simulink model "cubesatFullSim"  (R2024a)
settings: Solver=FixedStepAuto  StartTime=0.0  StopTime=20.0  FixedStep=0.1  MaxStep=1  MinStep=0.001  RelTol=1e-3
model workspace (MAT data in the model file):
  beta_initial = [0 0 0]
  com_quad_body = [1 0 0 0]
  imu_sample_time = 0.1
  initial_angular_momentum_body = [0 0 0]
  initial_datetime = [2020 3 17 23 48 32]
  initial_position_iss_orbit = [-2350000 -5230000 3530000]
  initial_quaterion_rotation = [0 0.7071 0.7071 0]
  initial_velocity_iss_orbit = [3990 -4820 -4820]
  intertia_tensor = [0.005743  -0.000107  -0.0006965; -0.000107  0.030927  8.6e-05; -0.000696  8.6e-05  0.030951]
  magnotorquer_current_to_magnetic = 1
  mass = 2.60014
  moi_spin_axis = 2.0292e-06
  onboard_att_ctrl_sample_time = 0.1
  onboard_att_det_sample_time = 0.1
  onboard_env_modelling_sample_time = 0.1
  q_n2m_initial = [1 0 0 0]
  reaction_wheel_state_space_A = [0  0  0  0; 0  0  0  0; 0  0  0  0; 0  0  0  0]
  reaction_wheel_state_space_B = [512  0  0  0; 0  512  0  0; 0  0  512  0; 0  0  0  512]
  reaction_wheel_state_space_C = [962.5  0  0  0; 0  962.5  0  0; 0  0  962.5  0; 0  0  0  962.5]
  reaction_wheel_state_space_D = [0  0  0  0; 0  0  0  0; 0  0  0  0; 0  0  0  0]
  reaction_wheel_state_space_initial = [0 0 0 0]
  steve_camera_axis_1 = [0 0 1]
  steve_camera_direction = [1 0 0]
libraries: vrlib x6
settings Model: Creator=samuel  LastModifiedBy=joshu
settings OptimizationCC: ReuseModelBlockBuffer=off
settings DebuggingCC: AlgebraicLoopMsg=error  ArtificialAlgebraicLoopMsg=error
settings ModelReferenceCC: EnableRefExpFcnMdlSchedulingChecks=on
settings RTWCC: GPUComputeCapability=3.5

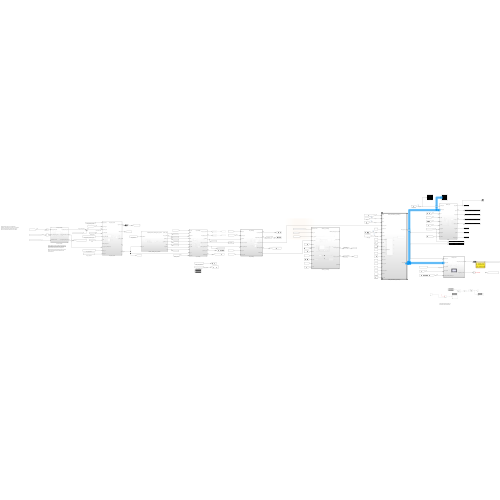
[thumbnail: Simulink's stored preview of the top-level diagram]
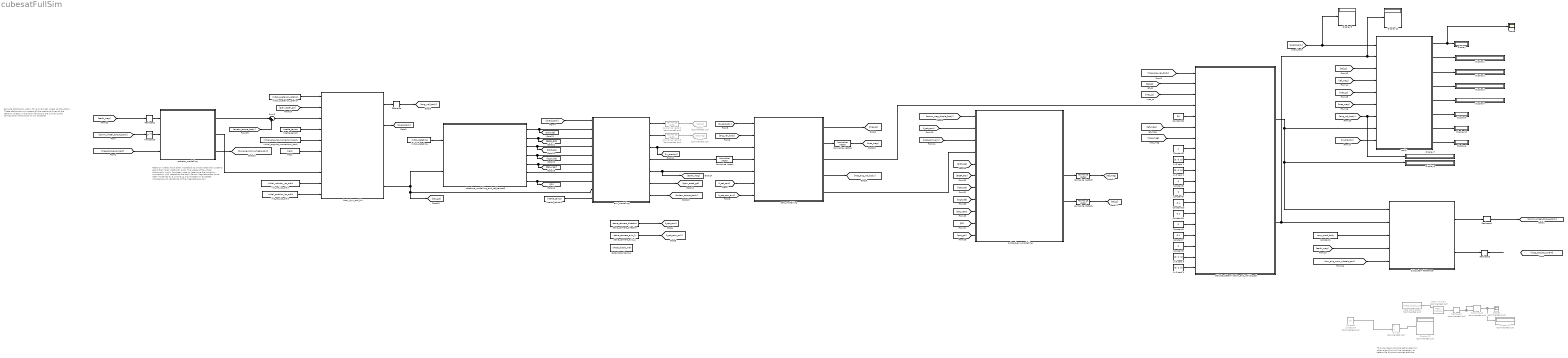
== system cubesatFullSim ==
  note: This provides a sample test quaternion, other algorithms will be necessary to determine this commanded attitude.
  note: Reaction wheels have been modelled as simple rotational systems about their local rotational axes. The usage of the wheel distribution matrix has been used to determine their angular momentum with respect to the body frame.
      |
      | Magnetorquers have been modelled as a simple LC circuit based on expected inductance and resistance of the magnetorquer coil.
  note: Sample distribution matrix for a pyramidal wheel configuration. These define the unit vectors of the rotational axes of the reaction wheels in the body frame and are similar to the configuration employed on our CubeSat.
  1x3 zero {1..4} (4 alike) : Constant  Value=[0, 0, 0]
  Constant : Constant  Commented=on  Value=2.0292e-6
  Constant1 : Constant  Value=com_quad_body
  Constant10 : Constant  Value=0.1
  Constant11 : Constant  Value=0.1
  Constant12 : Constant  Value=90
  Constant3 : Constant  OutDataTypeStr=boolean
  Constant5 : Constant  Value=0  OutDataTypeStr=boolean
  Constant6 : Constant  Value=0  OutDataTypeStr=boolean
  Constant7 : Constant  Value=0.1
  Constant8 : Constant  Value=0  OutDataTypeStr=boolean
  Constant9 : Constant  Value=0
  Data Store Memory : DataStoreMemory  DataStoreName=wheel_distrib_mat  WriteAfterWriteMsg=warning  InitialValue=[0.5736 0.5736 0.5736 0.5736 ; 0.8192 -0.8192 0 0 ; 0 0 0.8192 -0.8192]  ShowAdditionalParam=off
  Data Store Read1 : DataStoreRead  Commented=on  DataStoreName=wheel_distrib_mat  IndexOptions=Index vector (dialog)  Indices=1  OutputSizes=1
  Display{,1..11} (12 alike) : Display
  Display12 : Display  Commented=on
  Display13 : Display  Commented=on
  Divide : Product  Commented=on  Inputs=*/
  Dot Product : DotProduct  Commented=on  OutDataTypeStr=Inherit: Inherit via internal rule
  Goto7 : Goto  Commented=on  GotoTag=ref_ss
  Goto8 : Goto  Commented=on  GotoTag=ref_mag
  Matrix Multiply : Product  Commented=on  Multiplication=Matrix(*)
  Normalize Vector{,4..6} (4 alike) : vrlib/Utilities/Normalize Vector  maxzero=0
  Normalize Vector2 : vrlib/Utilities/Normalize Vector  Commented=on  maxzero=0
  Normalize Vector3 : vrlib/Utilities/Normalize Vector  Commented=on  maxzero=0
  Reshape : Reshape  OutputDimensionality=Row vector (2-D)
  Reshape1 : Reshape  OutputDimensionality=Row vector (2-D)
  Reshape2 : Reshape
  Reshape3 : Reshape
  Reshape5 : Reshape  Commented=on
  Scope : Scope
  Scope1 : Scope  Commented=on
  Subsystem Reference : Subsystem  TreatAsAtomicUnit=on  SystemSampleTime=onboard_att_ctrl_sample_time  ReferencedSubsystem=attitude_control
  Sum3 : Sum  Inputs=|++
  Transpose : Math  Operator=transpose
  Verify : Subsystem  ReferencedSubsystem=MEKF_verify
  actuator_modelling : Subsystem  ReferencedSubsystem=actuator_modelling
  attitude_determination_and_vehicle_est : Subsystem  TreatAsAtomicUnit=on  SystemSampleTime=onboard_att_det_sample_time  ReferencedSubsystem=attitude_determination_and_vehicle_est
      settings: PortSchema="{\"entries\":[{\"content\":{\"sides\":[{\"content\":{\"connectorIds\":[\"In1\",\"In2\",\"In3\",\"In4\",\"In15\",\"In5\",\"In6\",\"In7\",\"In8\",\"In9\",\"In10\",\"In11\",\"In12\",\"In13\",\"In14\",\"In16\",\"In17\",\"In18\",\"In19\"]},\"type\":\"ConnectorPlacement.EquallySpacedRectSide\",\"uuid\":\"3b22937b-158d-42bc-8266-221df4d5bb4f\"},{\"content\":{\"connectorIds\":[\"Out1\",\"Out2\"],\"side\":\"RIGHT\"},\"type\":\"ConnectorPlacement.EquallySpacedRectSide\",\"uuid\":\"2d7976b0-5d09-4ece-a5b5-6f5d6f0d46dd\"},{\"content\":{\"side\":\"TOP\"},\"type\":\"ConnectorPlacement.EquallySpacedRectSide\",\"uuid\":\"411abe81-91ab-4e83-a0ca-8600290f09f5\"}]},\"type\":\"ConnectorPlacement.EquallySpacedConnector\",\"uuid\":\"dff24d4c-a30b-41c1-92cc-a12930c50369\"}],\"packageUris\":[\"http://schema.mathworks.com/mf0/Connector/R2020b\"],\"version\":\"1.0\"}"
  body_dyn_and_kin : Subsystem  ReferencedSubsystem=body_dyn_and_kin
  datetime_modelling_and_ref_frames3 : Subsystem  ReferencedSubsystem=simplified_datetime_modelling_and_ref_frames
      settings: PortSchema="{\"entries\":[{\"content\":{\"sides\":[{\"content\":{\"connectorIds\":[\"In2\",\"In1\"]},\"type\":\"ConnectorPlacement.EquallySpacedRectSide\",\"uuid\":\"e6c4fb03-cad9-4384-b821-fab58a668bd5\"},{\"content\":{\"connectorIds\":[\"Out1\",\"Out2\",\"Out3\",\"Out4\",\"Out5\",\"Out6\",\"Out7\"],\"side\":\"RIGHT\"},\"type\":\"ConnectorPlacement.EquallySpacedRectSide\",\"uuid\":\"c6ed57d1-3bbe-4ef1-9925-a8ddf941e286\"},{\"content\":{\"side\":\"TOP\"},\"type\":\"ConnectorPlacement.EquallySpacedRectSide\",\"uuid\":\"f0e9b78b-8ccd-47fe-a025-ec59d36b78b7\"}]},\"type\":\"ConnectorPlacement.EquallySpacedConnector\",\"uuid\":\"673881b9-a40b-4646-b599-6ee2b2fc2b79\"}],\"packageUris\":[\"http://schema.mathworks.com/mf0/Connector/R2020b\"],\"version\":\"1.0\"}"
  env_modelling : Subsystem  ReferencedSubsystem=env_modelling
      settings: PortSchema="{\"entries\":[{\"content\":{\"sides\":[{\"content\":{\"connectorIds\":[\"In1\",\"In2\",\"In3\",\"In4\",\"In5\",\"In6\",\"In7\",\"In8\",\"In9\",\"In10\"]},\"type\":\"ConnectorPlacement.EquallySpacedRectSide\",\"uuid\":\"69fdfc0c-3415-4b98-a585-21dadab8ad42\"},{\"content\":{\"connectorIds\":[\"Out6\",\"Out5\",\"Out7\",\"Out4\",\"Out1\",\"Out2\",\"Out3\"],\"side\":\"RIGHT\"},\"type\":\"ConnectorPlacement.EquallySpacedRectSide\",\"uuid\":\"35c72ffa-2208-482d-8bc9-9a3522b3246b\"},{\"content\":{\"side\":\"TOP\"},\"type\":\"ConnectorPlacement.EquallySpacedRectSide\",\"uuid\":\"fd836a88-7f67-46c6-bc0e-0e53b2a2ba50\"}]},\"type\":\"ConnectorPlacement.EquallySpacedConnector\",\"uuid\":\"e74cc8e6-fb32-4c0f-8b27-d3f42cefd01b\"}],\"packageUris\":[\"http://schema.mathworks.com/mf0/Connector/R2020b\"],\"version\":\"1.0\"}"
  init_pos_iss_orbit : Constant  Value=initial_position_iss_orbit
  init_vel_iss_orbit : Constant  Value=initial_velocity_iss_orbit
  initial_angular_momentum_body : Constant  Value=initial_angular_momentum_body
  initial_datetime : Constant  Value=initial_datetime
  initial_quaterion_rotation : Constant  Value=initial_quaterion_rotation
  intertia_tensor : Constant  Value=intertia_tensor
  intertia_tensor1 : Constant  Value=intertia_tensor
  mass : Constant  Value=mass
  onboad_env_modelling : Subsystem  TreatAsAtomicUnit=on  SystemSampleTime=onboard_env_modelling_sample_time  ReferencedSubsystem=onboad_env_modelling
  sens_modelling : Subsystem  TreatAsAtomicUnit=on  ReferencedSubsystem=sens_modelling
      settings: PortSchema="{\"entries\":[{\"content\":{\"sides\":[{\"content\":{\"connectorIds\":[\"In4\",\"In3\",\"In7\",\"In2\",\"In1\",\"In5\",\"In6\"]},\"type\":\"ConnectorPlacement.EquallySpacedRectSide\",\"uuid\":\"1307c19a-9f54-4413-9c06-018e98633941\"},{\"content\":{\"connectorIds\":[\"Out2\",\"Out1\",\"Out5\",\"Out3\",\"Out4\"],\"side\":\"RIGHT\"},\"type\":\"ConnectorPlacement.EquallySpacedRectSide\",\"uuid\":\"4c634e96-4716-461b-adc9-f119018e3bb1\"},{\"content\":{\"side\":\"TOP\"},\"type\":\"ConnectorPlacement.EquallySpacedRectSide\",\"uuid\":\"0faf9cb0-e5fc-4cda-b249-42192f8504a8\"}]},\"type\":\"ConnectorPlacement.EquallySpacedConnector\",\"uuid\":\"414b1f49-1139-45d6-afb0-1a6007e1eaa7\"}],\"packageUris\":[\"http://schema.mathworks.com/mf0/Connector/R2020b\"],\"version\":\"1.0\"}"
  steve_camera_axis_1 : Constant  Value=steve_camera_axis_1
  steve_camera_direction : Constant  Value=steve_camera_direction
  wires:
  intertia_tensor/1 -> body_dyn_and_kin/4
  actuator_modelling/1 -> Sum3/1  "mag_act_torque_body"
  Sum3/1 -> body_dyn_and_kin/3  "tot_ext_mom_body"
  initial_angular_momentum_body/1 -> body_dyn_and_kin/5
  mass/1 -> body_dyn_and_kin/6
  actuator_modelling/2 -> body_dyn_and_kin/8
  init_vel_iss_orbit/1 -> body_dyn_and_kin/9
  init_pos_iss_orbit/1 -> body_dyn_and_kin/10
  attitude_determination_and_vehicle_est/1 -> Verify/8, Display8/1, Subsystem Reference/1
  attitude_determination_and_vehicle_est/2 -> Display11/1, Verify/2, Subsystem Reference/2  "meas_quat_body"
  Transpose/1 -> actuator_modelling/2
  Constant1/1 -> Subsystem Reference/3  "com_quat_body"
  Subsystem Reference/2 -> Reshape3/1
  [earth_mag] -> Reshape2/1
  sens_modelling/5 -> attitude_determination_and_vehicle_est/4
  1x3 zero 1/1 -> attitude_determination_and_vehicle_est/8
  1x3 zero 2/1 -> attitude_determination_and_vehicle_est/9
  Constant6/1 -> attitude_determination_and_vehicle_est/11
  Constant3/1 -> attitude_determination_and_vehicle_est/7
  Constant5/1 -> attitude_determination_and_vehicle_est/10
  Constant7/1 -> attitude_determination_and_vehicle_est/16
  Constant8/1 -> attitude_determination_and_vehicle_est/17
  Constant9/1 -> attitude_determination_and_vehicle_est/14
  Constant10/1 -> attitude_determination_and_vehicle_est/12
  Constant11/1 -> attitude_determination_and_vehicle_est/13
  1x3 zero 3/1 -> attitude_determination_and_vehicle_est/18
  1x3 zero 4/1 -> attitude_determination_and_vehicle_est/19
  initial_quaterion_rotation/1 -> body_dyn_and_kin/1
  body_dyn_and_kin/1 -> Reshape/1
  Subsystem Reference/1 -> Reshape1/1
  datetime_modelling_and_ref_frames3/6 -> env_modelling/7
  datetime_modelling_and_ref_frames3/2 -> [ECEF_GCI], env_modelling/3
  datetime_modelling_and_ref_frames3/3 -> [latitude], env_modelling/4
  datetime_modelling_and_ref_frames3/5 -> [dec_year], env_modelling/6
  datetime_modelling_and_ref_frames3/7 -> env_modelling/8, [JD]
  datetime_modelling_and_ref_frames3/1 -> [altitude], env_modelling/2
  datetime_modelling_and_ref_frames3/4 -> [logitude], env_modelling/5
  body_dyn_and_kin/5 -> datetime_modelling_and_ref_frames3/1, [pos_gci], env_modelling/9  "pos_gci"
  env_modelling/4 -> Normalize Vector/1
  [comm_wheel_torque_body] -> Transpose/1
  [mag_torquer_current] -> actuator_modelling/3
  [ang_vel_body] -> sens_modelling/3
  steve_camera_direction/1 -> [r_sat_com]
  steve_camera_axis_1/1 -> [r_sat_com_ax1]  "r_sat_com_ax1"
  [r_sat_com] -> sens_modelling/5
  [r_sat_com_ax1] -> sens_modelling/6
  sens_modelling/4 -> onboad_env_modelling/4
  [comm_mag_dipole_body] -> onboad_env_modelling/1
  [r_sat_com_ax1] -> onboad_env_modelling/3
  [r_sat_com] -> onboad_env_modelling/2
  env_modelling/6 -> Normalize Vector2/1
  Normalize Vector3/1 -> Goto8/1
  sens_modelling/1 -> Normalize Vector4/1
  Normalize Vector4/1 -> [mes_mag]
  sens_modelling/2 -> [mes_ss]
  body_dyn_and_kin/2 -> [quad_body]
  Reshape/1 -> [ang_vel_body]
  [mes_ang_vel_body] -> attitude_determination_and_vehicle_est/1
  Normalize Vector2/1 -> Goto7/1
  Constant12/1 -> attitude_determination_and_vehicle_est/15
  Normalize Vector/1 -> sens_modelling/2
  env_modelling/1 -> [earth_mag], sens_modelling/1
  env_modelling/7 -> [in_shadow], sens_modelling/7
  sens_modelling/3 -> [mes_ang_vel_body]
  [quad_body] -> Display5/1, Verify/1  "quad_body"
  [ang_vel_body] -> Verify/7, Display7/1
  [ref_ss] -> Verify/3
  [ref_mag] -> Verify/4
  [mes_ss] -> Verify/5
  [mes_mag] -> Verify/6
  Verify/1 -> Scope/1, Display/1
  Verify/2 -> Display1/1
  Verify/3 -> Display2/1
  Verify/4 -> Display3/1
  Verify/5 -> Display4/1
  Verify/8 -> Display6/1
  [in_shadow] -> Verify/9
  Verify/7 -> Display10/1
  Verify/6 -> Display9/1
  [mes_ss] -> attitude_determination_and_vehicle_est/3  "mes_ss"
  [mes_mag] -> attitude_determination_and_vehicle_est/6  "mes_mag"
  [ref_ss] -> attitude_determination_and_vehicle_est/2  "ref_ss"
  [ref_mag] -> attitude_determination_and_vehicle_est/5  "ref_mag"
  [quad_body] -> env_modelling/1
  [quad_body] -> sens_modelling/4
  env_modelling/2 -> [grav_accel_gci]
  env_modelling/3 -> [extern_torque_body]
  Reshape2/1 -> actuator_modelling/1
  [earth_mag] -> Subsystem Reference/4
  [grav_accel_gci] -> body_dyn_and_kin/2
  [extern_torque_body] -> Sum3/2
  actuator_modelling/3 -> [curr_ang_mom_wheels_spin]
  env_modelling/5 -> Normalize Vector3/1
  Reshape3/1 -> ?
  Data Store Read1/1 -> Matrix Multiply/1
  Matrix Multiply/1 -> Reshape5/1
  Dot Product/1 -> Display13/1, Scope1/1
  Reshape5/1 -> Dot Product/1, Dot Product/2
  Constant/1 -> Divide/2
  Divide/1 -> Display12/1
  initial_datetime/1 -> datetime_modelling_and_ref_frames3/2
  [JD] -> onboad_env_modelling/10
  [logitude] -> onboad_env_modelling/8
  [dec_year] -> onboad_env_modelling/9
  [pos_gci] -> onboad_env_modelling/11
  [latitude] -> onboad_env_modelling/7
  [ECEF_GCI] -> onboad_env_modelling/6
  [altitude] -> onboad_env_modelling/5
  intertia_tensor1/1 -> env_modelling/10
  [curr_ang_mom_wheels_spin] -> Subsystem Reference/5
  ? -> Divide/1
  onboad_env_modelling/3 -> Normalize Vector5/1
  onboad_env_modelling/4 -> Normalize Vector6/1
  Normalize Vector6/1 -> [ref_ss]
  Normalize Vector5/1 -> [ref_mag]
  Reshape1/1 -> [comm_wheel_torque_body]
